simulink model "Sl_blind_object_NelineinaSistema_SIMULATION"  (R2015a)
settings: Solver=ode15s  StartTime=0.0  StopTime=2000  RelTol=1e-3
values from neighbouring files (symbols this model uses):
  J = 1    [Sc_blind_object.m]
  kedn = 100    [Sc_blind_object.m]
  kl = 1    [Sc_blind_object.m]
  km = 1    [Sc_blind_object.m]
  kt = 10    [Sc_blind_object.m]
  L = 1    [Sc_blind_object.m]
  R = 100    [Sc_blind_object.m]
  T = 1    [Sc_blind_object.m]
libraries: cstblocks x1
settings Model: Creator=Vladislav  LastModifiedBy=Vladislav

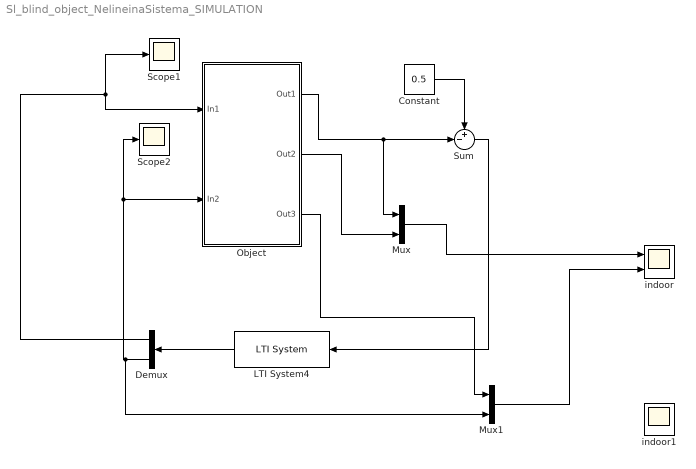
== system Sl_blind_object_NelineinaSistema_SIMULATION ==
  Constant : Constant  Value=0.5
  Demux : Demux  Outputs=2
  LTI System4 : cstblocks/LTI System  sys=K  IC=[]
  Mux : Mux  Inputs=2
  Mux1 : Mux  Inputs=2
  Object : Subsystem
  Scope1 : Scope
      settings: YMin=0.066  YMax=0.08  SaveName=ScopeData4
  Scope2 : Scope
      settings: YMin=1.2  YMax=2  SaveName=ScopeData5
  Sum : Sum  Inputs=+-|
  indoor : Scope  NumInputPorts=2
      settings: TimeRange=100  YMin=-0.5~-5  YMax=2.77556e-17~5
  indoor1 : Scope
      settings: TimeRange=100  YMin=-0.5  YMax=2.775557561562891e-17  SaveName=ScopeData6
  wires:
  Demux/1 -> Object/1(In1), Scope1/1
  Object/1(Out1) -> Mux/1, Sum/2
  LTI System4/1 -> Demux/1
  Sum/1 -> LTI System4/1
  Constant/1 -> Sum/1
  Demux/2 -> Mux1/2, Scope2/1, Object/2(In2)
  Object/2(Out2) -> Mux/2
  Mux/1 -> indoor/1
  Object/3(Out3) -> Mux1/1
  Mux1/1 -> indoor/2

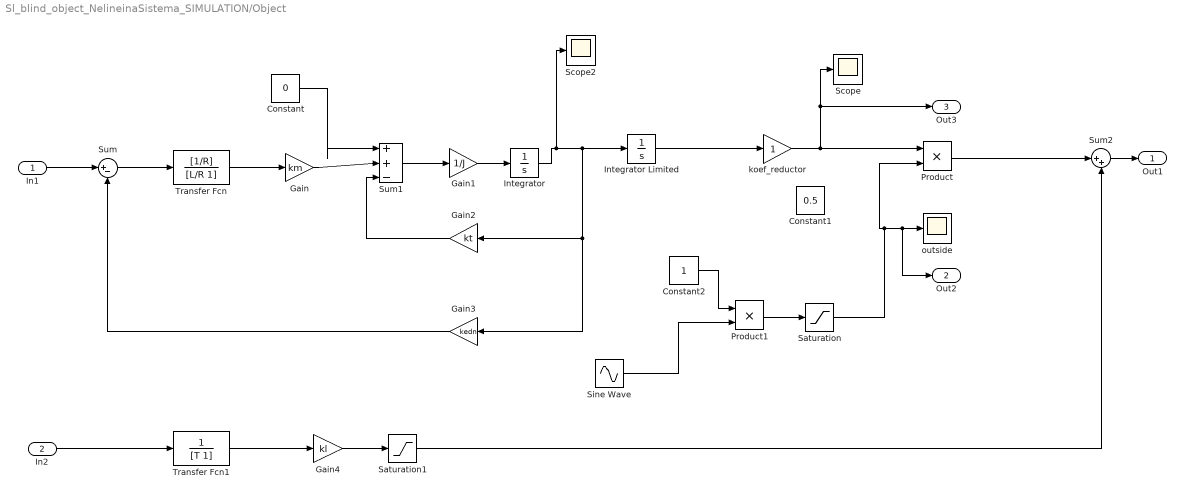
== system Sl_blind_object_NelineinaSistema_SIMULATION/Object ==
  In1 : Inport
  In2 : Inport  Port=2
  Constant : Constant  Value=0
  Constant1 : Constant  Value=0.5
  Constant2 : Constant
  Gain : Gain  Gain=km
  Gain1 : Gain  Gain=1/J
  Gain2 : Gain  Gain=kt
  Gain3 : Gain  Gain=kedn
  Gain4 : Gain  Gain=kl
  Integrator : Integrator
  Integrator Limited : Integrator  LimitOutput=on  UpperSaturationLimit=1  LowerSaturationLimit=0  IgnoreLimit=on
  Product : Product
  Product1 : Product
  Saturation : Saturate  UpperLimit=Inf  LowerLimit=0
  Saturation1 : Saturate  UpperLimit=1  LowerLimit=0
  Scope : Scope
  Scope2 : Scope
      settings: SaveName=ScopeData3
  Sine Wave : Sin  Amplitude=0.5  Bias=0.5  Frequency=1/1440*2*pi  SampleTime=0
  Sum : Sum  Inputs=|+-
  Sum1 : Sum  Inputs=|++-
  Sum2 : Sum  Inputs=|++
  Transfer Fcn : TransferFcn  Numerator=[1/R]  Denominator=[L/R 1]
  Transfer Fcn1 : TransferFcn  Denominator=[T 1]
  koef_reductor : Gain
  outside : Scope
      settings: SaveName=ScopeData2
  Out1 : Outport
  Out2 : Outport  Port=2
  Out3 : Outport  Port=3
  wires:
  Transfer Fcn/1 -> Gain/1
  In2/1 -> Transfer Fcn1/1
  Product1/1 -> Saturation/1
  Sum/1 -> Transfer Fcn/1
  Sum1/1 -> Gain1/1
  Gain1/1 -> Integrator/1
  koef_reductor/1 -> Product/1, Out3/1, Scope/1
  In1/1 -> Sum/1
  Gain/1 -> Sum1/2
  Constant/1 -> Sum1/1
  Integrator Limited/1 -> koef_reductor/1
  Gain3/1 -> Sum/2
  Gain2/1 -> Sum1/3
  Product/1 -> Sum2/1
  Integrator/1 -> Scope2/1, Gain3/1, Gain2/1, Integrator Limited/1
  Sine Wave/1 -> Product1/2
  Saturation/1 -> Product/2, Out2/1, outside/1
  Transfer Fcn1/1 -> Gain4/1
  Sum2/1 -> Out1/1
  Gain4/1 -> Saturation1/1
  Constant2/1 -> Product1/1
  Saturation1/1 -> Sum2/2
